simulink model "SinglePulseN4"  (R2014b)
settings: Solver=ode45  StartTime=0.0  StopTime=10.0  RelTol=1e-3
PreLoadFcn:
  | initialize;
undefined symbols (not defined in the file or in its folder): inputSequence
libraries: BlockLib x11, dspsrcs4 x1
settings Model: Creator=lstmarie  LastModifiedBy=kunalmenda
settings DebuggingCC: UnderspecifiedInitializationDetection=Classic  MergeDetectMultiDrivingBlocksExec=none

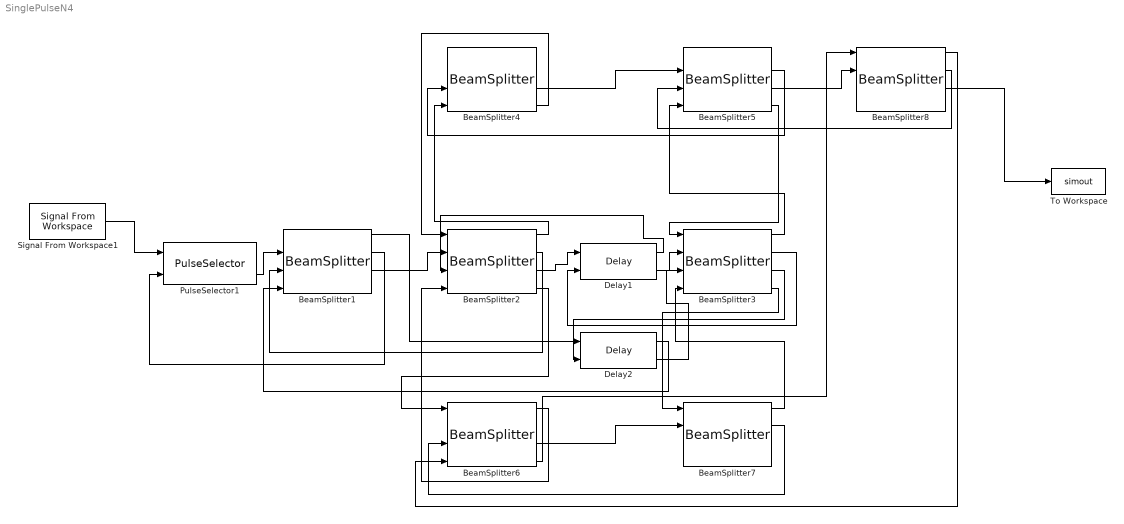
== system SinglePulseN4 ==
  BeamSplitter{1..8} (8 alike) : BlockLib/BeamSplitter  Transmittance=0.50  Reflectance=0.50  Ghost=0.01  BackReflectance=0.001
  Delay1 : BlockLib/Delay  DelayAmt=10e-9
  Delay2 : BlockLib/Delay  DelayAmt=10e-9
  PulseSelector1 : BlockLib/PulseSelector  PCTimings=[-1,1,38,40,103,105,168,170,220,274]*1e-9  ControlPowers=[0.5000, 1.0000,1.0000, 1.0000, 0.5000]
  Signal From Workspace1 : dspsrcs4/Signal From Workspace  X=inputSequence(13*10^-9,1,0,130*10^-9)  Ts=1  nsamps=1  OutputAfterFinalValue=Setting to zero  ignoreOrWarnInputAndFrameLengths=off
  To Workspace : ToWorkspace  VariableName=simout  SaveFormat=Timeseries  SampleTime=-1
  wires:
  Signal From Workspace1/1 -> PulseSelector1/1
  BeamSplitter8/3 -> To Workspace/1
  BeamSplitter1/1 -> Delay2/1
  BeamSplitter2/1 -> BeamSplitter4/4
  BeamSplitter1/3 -> BeamSplitter2/2
  BeamSplitter2/3 -> Delay1/1
  BeamSplitter2/4 -> BeamSplitter6/1
  Delay1/2 -> BeamSplitter3/2
  BeamSplitter3/1 -> BeamSplitter5/4
  BeamSplitter3/3 -> Delay2/2
  BeamSplitter2/2 -> BeamSplitter1/3
  BeamSplitter1/2 -> PulseSelector1/2
  Delay1/1 -> BeamSplitter2/3
  BeamSplitter4/4 -> BeamSplitter2/1
  BeamSplitter3/2 -> Delay1/2
  BeamSplitter4/3 -> BeamSplitter5/2
  BeamSplitter5/2 -> BeamSplitter4/3
  BeamSplitter6/1 -> BeamSplitter2/4
  Delay2/1 -> BeamSplitter1/4
  BeamSplitter7/2 -> BeamSplitter6/3
  BeamSplitter8/1 -> BeamSplitter6/4
  BeamSplitter6/3 -> BeamSplitter7/2
  BeamSplitter6/4 -> BeamSplitter8/1
  BeamSplitter3/4 -> BeamSplitter7/1
  BeamSplitter7/1 -> BeamSplitter3/4
  Delay2/2 -> BeamSplitter3/3
  BeamSplitter5/4 -> BeamSplitter3/1
  BeamSplitter8/2 -> BeamSplitter5/3
  BeamSplitter5/3 -> BeamSplitter8/2
  PulseSelector1/2 -> BeamSplitter1/2
